simulink model "ctrld_4Q_Chopper"  (R2023b)
settings: Solver=ode45  StartTime=0.0  StopTime=0.1  MaxStep=1e-3  RelTol=1e-4
values from neighbouring files (symbols this model uses):
  E = 0    [TP_Hacheurs.m]
  L = 0.1    [TP_Hacheurs.m]
  R = 10    [TP_Hacheurs.m]
  T = 1/f    (= 0.002)    [TP_Hacheurs.m]
  U_Reference = -14    [TP_Hacheurs.m]
  Vdc = 50    [TP_Hacheurs.m]
libraries: spsIGBTDiodeLib x4, spsDCVoltageSourceLib x3, spsMeanLib x2, simulink x1, spsCurrentMeasurementLib x1, spsSeriesRLCBranchLib x1, spsVoltageMeasurementLib x1, sps_lib x1
settings Model: Creator=Legrey  LastModifiedBy=Legrey

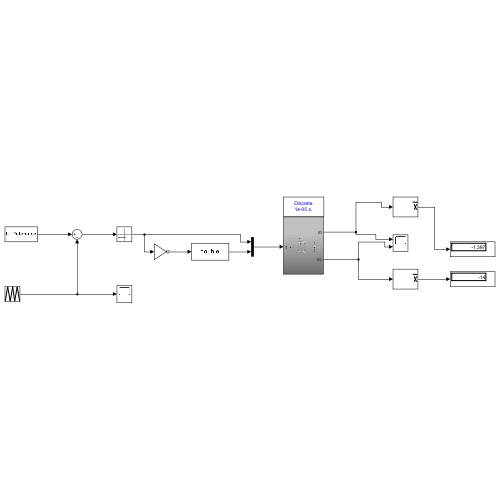
[thumbnail: Simulink's stored preview of the top-level diagram]
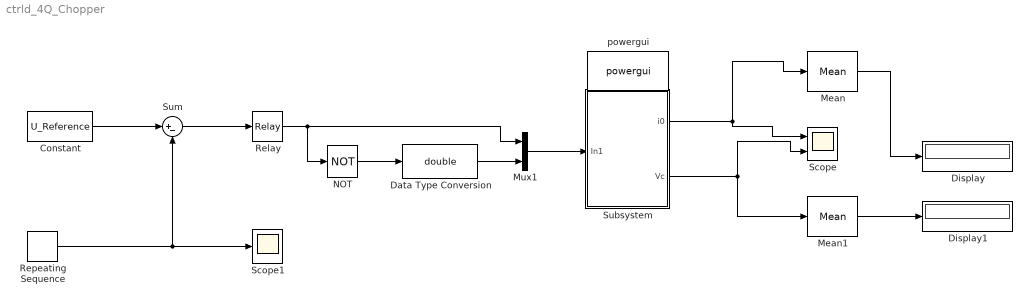
== system ctrld_4Q_Chopper ==
  Constant : Constant  Value=U_Reference
  Data Type Conversion : DataTypeConversion  OutDataTypeStr=double  SaturateOnIntegerOverflow=off  RndMeth=Floor
  Display : Display
  Display1 : Display
  Mean : spsMeanLib/Mean  Freq=f  Vinit=0  Ts=0
  Mean1 : spsMeanLib/Mean  Freq=f  Vinit=0  Ts=0
  Mux1 : Mux  Inputs=2
  NOT : Logic  Operator=NOT  IconShape=distinctive  AllPortsSameDT=off  OutDataTypeStr=boolean
  Relay : Relay  OnSwitchValue=0  OffSwitchValue=0
  Repeating Sequence : simulink/Sources/Repeating Sequence  rep_seq_t=[0 1/2 1]*T  rep_seq_y=[-Vdc Vdc -Vdc]
  Scope : Scope  NumInputPorts=2
  Scope1 : Scope
  Subsystem : Subsystem
  Sum : Sum  Inputs=|+-
  powergui : sps_lib/powergui  Priority=1  SimulationMode=Discrete  SampleTime=1e-005  frequency=60  Iterations=50  frequencyindice=0  Pbase=100e6  ErrMax=1e-4  UnitsV=kV  UnitsW=MW  buscounter=0  FunctionMessages=off  echomessages=off  EnableUseOfTLC=off  CurrentSourceSwitches=off  DisableSnubberDevices=off  DisableRonSwitches=off  DisableVfSwitches=off  DisplayEquations=off  AutomaticDiscreteSolvers=off  SolverType=Tustin/Backward Euler (TBE)  Interpol=off  ExternalGateDelay=off  methode=off  Ts=100  x0status=blocks  SPID=on  SwTol=0  HookPort=off  NonlinearTolerance=1e-4  nMaxIteration=100  ContinueOnMaxIteration=off  RestoreLinks=warning  ResistiveCurrentMeasurement=off  Frange=[0:2:500]  Ylog=off  Xlog=on  ShowGrid=off  save=off  variable=ZData  structure=0  ZoomFFT=off  StartTime=0.0  cycles=1  DisplayStyle=1  fundamental=60  FreqAxis=off  MaxFrequency=1000  frequencyindicesteady=1  RmsSteady=1  display=off
  wires:
  Sum/1 -> Relay/1
  Repeating Sequence/1 -> Sum/2, Scope1/1
  Constant/1 -> Sum/1
  Subsystem/2(Vc) -> Scope/2, Mean1/1
  Mean1/1 -> Display1/1
  Mean/1 -> Display/1
  Subsystem/1(i0) -> Mean/1, Scope/1
  Mux1/1 -> Subsystem/1(In1)
  Data Type Conversion/1 -> Mux1/2
  NOT/1 -> Data Type Conversion/1
  Relay/1 -> Mux1/1, NOT/1

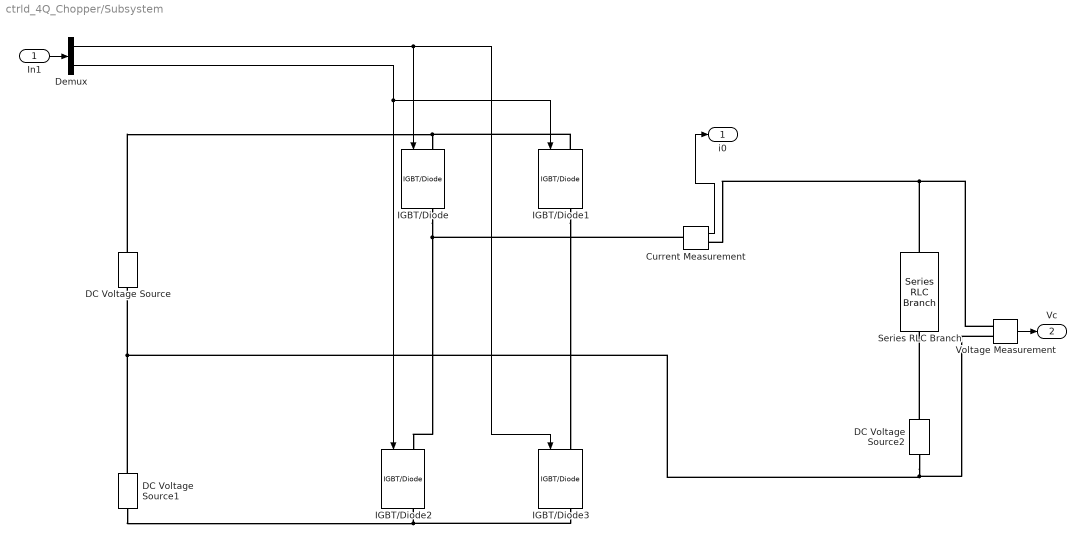
== system ctrld_4Q_Chopper/Subsystem ==
  In1 : Inport
  Current Measurement : spsCurrentMeasurementLib/Current Measurement  PhasorSimulation=off  OutputType=Complex  PSBequivalent=0
  DC Voltage Source : spsDCVoltageSourceLib/DC Voltage Source  Amplitude=Vdc  Measurements=None
  DC Voltage Source1 : spsDCVoltageSourceLib/DC Voltage Source  Amplitude=Vdc  Measurements=None
  DC Voltage Source2 : spsDCVoltageSourceLib/DC Voltage Source  Amplitude=E  Measurements=None
  Demux : Demux  Outputs=2
  IGBT/Diode{,1..3} (4 alike) : spsIGBTDiodeLib/IGBT//Diode  Ron=1e-3  Rs=1e5  Cs=inf  Measurements=on
  Series RLC Branch : spsSeriesRLCBranchLib/Series RLC Branch  LConnTagsString=__new0  RConnTagsString=__new0  BranchType=RL  Resistance=R  Inductance=L  SetiL0=off  InitialCurrent=0  Capacitance=1e-6  Setx0=off  InitialVoltage=0  Measurements=None
  Voltage Measurement : spsVoltageMeasurementLib/Voltage Measurement  PhasorSimulation=off  OutputType=Complex  PSBequivalent=0
  i0 : Outport
  Vc : Outport  Port=2
  wires:
  Voltage Measurement/1 -> Vc/1
  In1/1 -> Demux/1
  Demux/2 -> IGBT/Diode1/1, IGBT/Diode2/1
  Demux/1 -> IGBT/Diode3/1, IGBT/Diode/1
  Current Measurement/1 -> i0/1
  connections:
  DC Voltage Source/RConn1 -- IGBT/Diode1/LConn1 -- IGBT/Diode/LConn1
  DC Voltage Source1/RConn1 -- Voltage Measurement/LConn2 -- DC Voltage Source2/LConn1 -- DC Voltage Source/LConn1
  IGBT/Diode/RConn1 -- Current Measurement/LConn1 -- IGBT/Diode2/LConn1
  Series RLC Branch/LConn1 -- Current Measurement/RConn1 -- Voltage Measurement/LConn1
  DC Voltage Source2/RConn1 -- Series RLC Branch/RConn1
  DC Voltage Source1/LConn1 -- IGBT/Diode3/RConn1 -- IGBT/Diode2/RConn1
  IGBT/Diode1/RConn1 -- IGBT/Diode3/LConn1
